simulink model "Brakesimulation"  (R2023b)
settings: Solver=VariableStepAuto  StartTime=0.0  StopTime=300  RelTol=1e-3
InitFcn:
  | g=9.81; %32.18;
  | v0=120/3.6; %88;
  | Rr=0.45; % Wheel radius
  | Kf=1;
  | m=1000; %50;
  | PBmax=1500;
  | TB=0.01;
  | I=5;
  | %
  | % Mu slip curve
  | %
  | slip=[0 : 0.05 : 1.0];
  | mu=[0 0.4 0.8 0.97 1 0.98 0.96 0.94 0.92 0.9 0.88 0.855 0.83 0.81 0.79 0.77 0.75 0.73 0.72 0.71 0.7];
  | ctrl=1;
settings Model: Creator=김준현  LastModifiedBy=김준현

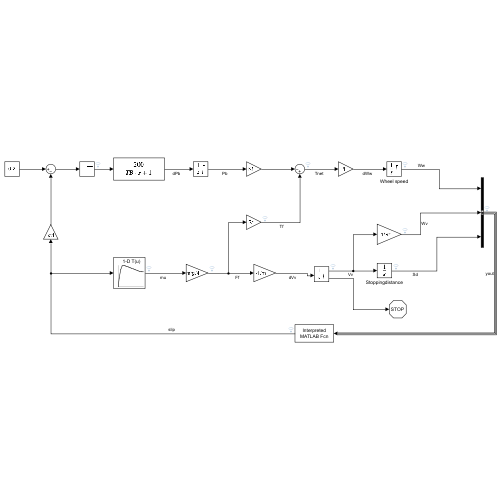
[thumbnail: Simulink's stored preview of the top-level diagram]
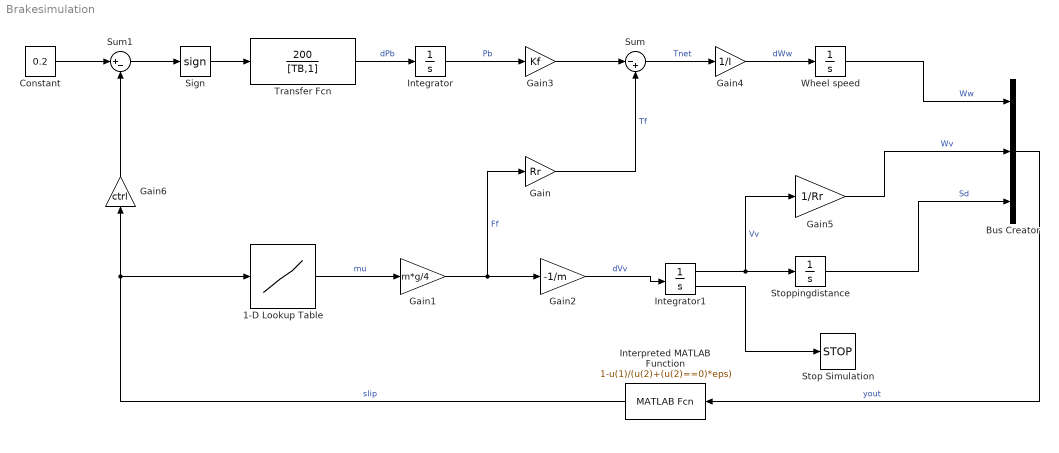
== system Brakesimulation ==
  1-D Lookup Table : Lookup_n-D  NumberOfTableDimensions=1  BreakpointsForDimension1=slip  Table=mu  InternalRulePriority=Speed  RndMeth=Simplest
  Bus Creator : BusCreator  Inputs=3
  Constant : Constant  Value=0.2
  Gain : Gain  Gain=Rr
  Gain1 : Gain  Gain=m*g/4
  Gain2 : Gain  Gain=-1/m
  Gain3 : Gain  Gain=Kf
  Gain4 : Gain  Gain=1/I
  Gain5 : Gain  Gain=1/Rr
  Gain6 : Gain  Gain=ctrl
  Integrator : Integrator  LimitOutput=on  UpperSaturationLimit=1500  LowerSaturationLimit=0
  Integrator1 : Integrator  InitialCondition=v0  LimitOutput=on  UpperSaturationLimit=1000  LowerSaturationLimit=0  ShowSaturationPort=on
  Interpreted MATLAB Function : MATLABFcn  MATLABFcn=1-u(1)/(u(2)+(u(2)==0)*eps)  OutputDimensions=1
  Sign : Signum
  Stop Simulation : Stop
  Stoppingdistance : Integrator
  Sum : Sum  Inputs=|-+
  Sum1 : Sum  Inputs=|+-
  Transfer Fcn : TransferFcn  Numerator=200  Denominator=[TB,1]
  Wheel speed : Integrator  InitialCondition=v0/Rr  LimitOutput=on  UpperSaturationLimit=1000  LowerSaturationLimit=0
  wires:
  Gain1/1 -> Gain/1, Gain2/1  "Ff"
  Gain/1 -> Sum/2  "Tf"
  Gain2/1 -> Integrator1/1  "dVv"
  Integrator/1 -> Gain3/1  "Pb"
  Gain3/1 -> Sum/1
  Sum/1 -> Gain4/1  "Tnet"
  Gain4/1 -> Wheel speed/1  "dWw"
  Transfer Fcn/1 -> Integrator/1  "dPb"
  Wheel speed/1 -> Bus Creator/1  "Ww"
  Integrator1/1 -> Stoppingdistance/1, Gain5/1  "Vv"
  Gain5/1 -> Bus Creator/2  "Wv"
  Stoppingdistance/1 -> Bus Creator/3  "Sd"
  Bus Creator/1 -> Interpreted MATLAB Function/1  "yout"
  Interpreted MATLAB Function/1 -> 1-D Lookup Table/1, Gain6/1  "slip"
  1-D Lookup Table/1 -> Gain1/1  "mu"
  Gain6/1 -> Sum1/2
  Constant/1 -> Sum1/1
  Sum1/1 -> Sign/1
  Sign/1 -> Transfer Fcn/1
  Integrator1/2 -> Stop Simulation/1
